simulink model "Torque_Control_ETR07"  (R2017b)
settings: Solver=FixedStepAuto  StartTime=0.0  StopTime=10.0  RelTol=1e-3
libraries: simulink x15, dspstat3 x1
(part 1 of 5)
settings Model: Creator=cspt  LastModifiedBy=cspt
settings RTWCC: SystemTargetFile=irt.tlc  TemplateMakefile=irt_default_tmf  Description=INTECRIO Real-Time Target
settings STFCustomTargetCC: TargetLangStandard=C99 (ISO)  UtilityFuncGeneration=Shared location  SystemTargetFile=irt.tlc
settings GRTTargetCC: UtilityFuncGeneration=Shared location  ParMdlRefBuildCompliant=off  CompOptLevelCompliant=off  ConcurrentExecutionCompliant=off  CombineOutputUpdateFcns=off  MatFileLogging=off  CPPClassGenCompliant=off  GRTInterface=on  UseToolchainInfoCompliant=off  GenerateASAP2=on

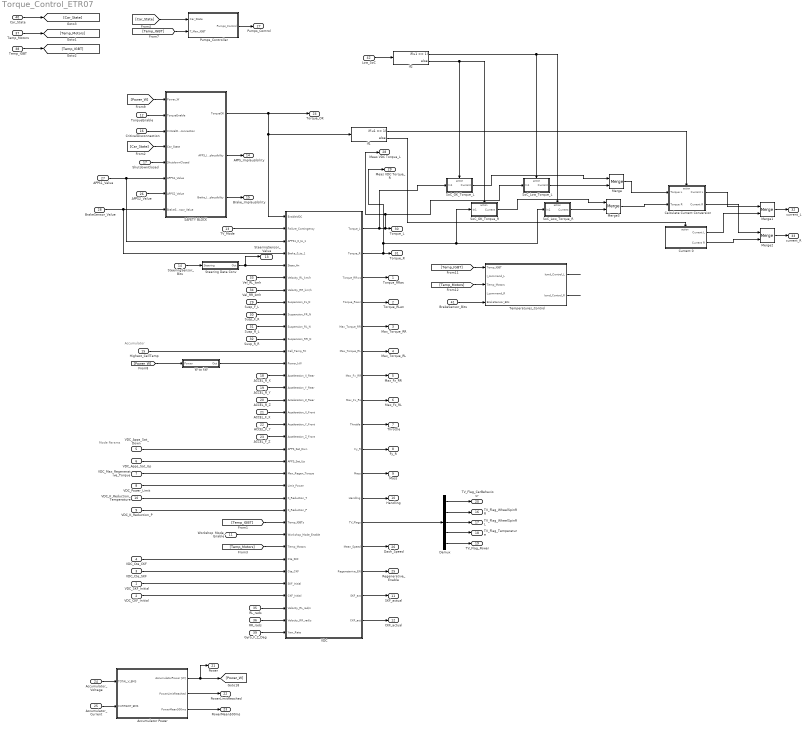
== system Torque_Control_ETR07 ==
  note: Mode Params
  note: Accumulator
  VDC_SKF_Initial : Inport
  VDC_CKF_Initial : Inport  Port=2
  VDC_Cte_SKF : Inport  Port=3
  VDC_Cte_CKF : Inport  Port=4
  VDC_Apps_Sat_Down : Inport  Port=5
  VDC_Apps_Sat_Up : Inport  Port=6
  VDC_Max_Regenerative_Torque : Inport  Port=7
  VDC_Power_Limit : Inport  Port=8
  VDC_K_Reduction_P : Inport  Port=9
  VDC_K_Reduction_Temperature : Inport  Port=10
  Workshop_Mode_Enable : Inport  Port=11
  TorqueEnable : Inport  Port=12
  TV_Mode : Inport  Port=13
  SteeringSensor_Bits : Inport  Port=14
  Highest_CellTemp : Inport  Port=15
  CriticalDisconnection : Inport  Port=16
  ShutdownClosed : Inport  Port=17
  ACCEL_R_X : Inport  Port=18
  ACCEL_R_Y : Inport  Port=19
  ACCEL_R_Z : Inport  Port=20
  ACCEL_F_X : Inport  Port=21
  ACCEL_F_Y : Inport  Port=22
  ACCEL_F_Z : Inport  Port=23
  Accumulator_Voltage : Inport  Port=24
  Accumulator_Current : Inport  Port=25
  APPS2_Value : Inport  Port=26
  APPS1_Value : Inport  Port=27
  BrakeSensor_Value : Inport  Port=28
  Susp_F_L : Inport  Port=29
  Susp_F_R : Inport  Port=30
  Susp_R_L : Inport  Port=31
  Susp_R_R : Inport  Port=32
  Vel_RL_kmh : Inport  Port=33
  Vel_RR_kmh : Inport  Port=34
  RL_rads : Inport  Port=35
  RR_rads : Inport  Port=36
  Temp_Motors : Inport  Port=37
  Temp_IGBT : Inport  Port=38
  Gyro_F_Z_Deg : Inport  Port=39
  Car_State : Inport  Port=40
  BrakeSensor_Bits : Inport  Port=41
  Low_SoC : Inport  Port=42
  Accumulator Power : Subsystem
  Calculate Current Conversion : Subsystem
  Current 0 : Subsystem  TreatAsAtomicUnit=on
  Demux : Demux  Outputs=5
  If1 : If  IfExpression=u1 == 1
  If2 : If  IfExpression=u1 == 1
  Merge{,1..3} (4 alike) : Merge
  Pumps_Controller : Subsystem
  SAFETY BLOCK : Subsystem
  SoC_Low_Torque_L : Subsystem  TreatAsAtomicUnit=on
  SoC_Low_Torque_R : Subsystem  TreatAsAtomicUnit=on
  SoC_OK_Torque_L : Subsystem  TreatAsAtomicUnit=on
  SoC_OK_Torque_R : Subsystem  TreatAsAtomicUnit=on
  Steering Data Conv : Subsystem
  Temperatures_Control : Subsystem
  VDC : Subsystem
  W to kW : Subsystem
  Torque_RRwc : Outport
  Torque_RLwc : Outport  Port=2
  Max_Torque_RR : Outport  Port=3
  Max_Torque_RL : Outport  Port=4
  Max_Fx_RR : Outport  Port=5
  Max_Fx_RL : Outport  Port=6
  Throttle : Outport  Port=7
  Fy_R : Outport  Port=8
  Mass : Outport  Port=9
  Handling : Outport  Port=10
  SKF_actual : Outport  Port=11
  CKF_actual : Outport  Port=12
  SteeringSensor_Value : Outport  Port=13
  APPS_Implausibility : Outport  Port=14
  Brake_Implausibility : Outport  Port=15
  TV_Flag_WheelSpinRR : Outport  Port=16
  TV_Flag_WheelSpinRL : Outport  Port=17
  TV_Flag_Temperature : Outport  Port=18
  TV_Flag_Power : Outport  Port=19
  TV_Flag_CarBehaviour : Outport  Port=20
  Power : Outport  Port=21
  PowerLimitReached : Outport  Port=22
  PowerMean500ms : Outport  Port=23
  Torque_OK : Outport  Port=24
  Regenerative_Enable : Outport  Port=25
  Dash_Speed : Outport  Port=26
  Pumps_Control : Outport  Port=27
  Meas VDC Torque_L : Outport  Port=28
  Meas VDC Torque_R : Outport  Port=29
  Torque_L : Outport  Port=30
  Torque_R : Outport  Port=31
  current_L : Outport  Port=32
  current_R : Outport  Port=33
  wires:
  Current 0/2(Current R) -> Merge2/2
  Accumulator Power/1(AccumulatorPower [W]) -> [Power_W], Power/1
  VDC_K_Reduction_P/1 -> VDC/25(K_Reduction_P)
  Workshop_Mode_Enable/1 -> VDC/27(Workshop_Mode_Enable)
  SAFETY BLOCK/2(APPS_Implausibility) -> APPS_Implausibility/1
  VDC_Cte_SKF/1 -> VDC/30(Cte_CKF)
  Calculate Current Conversion/2(Current R) -> Merge2/1
  Demux/4 -> TV_Flag_Temperature/1
  VDC_Apps_Sat_Down/1 -> VDC/20(APPS_Sat_Dwn)
  VDC_Max_Regenerative_Torque/1 -> VDC/22(Max_Regen_Torque)
  VDC_K_Reduction_Temperature/1 -> VDC/24(K_Reduction_T)
  VDC_Power_Limit/1 -> VDC/23(Limit_Power)
  VDC_Cte_CKF/1 -> VDC/29(Cte_SKF)
  VDC_SKF_Initial/1 -> VDC/31(SKF_Initial)
  VDC/2(Torque_R) -> SoC_OK_Torque_R/1(In1), SoC_Low_Torque_R/1(In1), Meas VDC Torque_R/1, Torque_R/1
  VDC/3(Torque_RRwc) -> Torque_RRwc/1
  TV_Mode/1 -> VDC/2(Failure_Contingency)
  W to kW/1(Out) -> VDC/13(Power_kW)
  Highest_CellTemp/1 -> VDC/12(Cell_Temp_ºC)
  ACCEL_F_X/1 -> VDC/17(Acceleration_X_Front)
  [Car_State] -> SAFETY BLOCK/4(Car_State)
  ACCEL_R_X/1 -> VDC/14(Acceleration_X_Rear)
  Accumulator_Current/1 -> Accumulator Power/2(CURRENT_BMS)
  Accumulator Power/3(PowerMean500ms) -> PowerMean500ms/1
  SteeringSensor_Bits/1 -> Steering Data Conv/1("Steering ")
  [Temp_Motors] -> VDC/28(Temp_Motors)
  [Temp_IGBT] -> Pumps_Controller/2(T_Max_IGBT)
  VDC/14(Mean_Speed) -> Dash_Speed/1
  Pumps_Controller/1(Pumps_Control) -> Pumps_Control/1
  Demux/1 -> TV_Flag_CarBehaviour/1
  VDC/15(Regenetarive_EN) -> Regenerative_Enable/1
  VDC/10(Fy_R) -> Fy_R/1
  Current 0/1(Current L) -> Merge1/2
  Calculate Current Conversion/1(Current L) -> Merge1/1
  If1/2 -> Current 0/Action
  If1/1 -> Calculate Current Conversion/Action
  VDC_Apps_Sat_Up/1 -> VDC/21(APPS_Sat_Up)
  TorqueEnable/1 -> SAFETY BLOCK/2(TorqueEnable)
  VDC/5(Max_Torque_RR) -> Max_Torque_RR/1
  Accumulator_Voltage/1 -> Accumulator Power/1(TOTAL_V_BMS)
  Accumulator Power/2(PowerLimitReached) -> PowerLimitReached/1
  VDC/7(Max_Fx_RR) -> Max_Fx_RR/1
  VDC/8(Max_Fx_RL) -> Max_Fx_RL/1
  VDC_CKF_Initial/1 -> VDC/32(CKF_Initial)
  SAFETY BLOCK/3(Brake_Implausibility) -> Brake_Implausibility/1
  Demux/2 -> TV_Flag_WheelSpinRR/1
  ACCEL_R_Y/1 -> VDC/15(Acceleration_Y_Rear)
  ACCEL_R_Z/1 -> VDC/16(Acceleration_Z_Rear)
  Demux/5 -> TV_Flag_Power/1
  VDC/9(Throttle) -> Throttle/1
  Demux/3 -> TV_Flag_WheelSpinRL/1
  ACCEL_F_Z/1 -> VDC/19(Acceleration_Z_Front)
  [Power_W] -> W to kW/1(Power)
  [Temp_IGBT] -> VDC/26(Temp_IGBTs)
  ACCEL_F_Y/1 -> VDC/18(Acceleration_Y_Front)
  CriticalDisconnection/1 -> SAFETY BLOCK/3(CriticalDisconnection)
  SAFETY BLOCK/1(TorqueOK) -> Torque_OK/1, VDC/1(EnableVDC), If1/1
  ShutdownClosed/1 -> SAFETY BLOCK/5(ShutdownClosed)
  VDC/11(Mass) -> Mass/1
  VDC/17(CKF_act) -> CKF_actual/1
  VDC/12(Handling) -> Handling/1
  VDC/13(TV_Flags) -> Demux/1
  VDC/6(Max_Torque_RL) -> Max_Torque_RL/1
  VDC/16(SKF_act) -> SKF_actual/1
  [Power_W] -> SAFETY BLOCK/1(Power_W)
  VDC/4(Torque_RLwc) -> Torque_RLwc/1
  APPS1_Value/1 -> SAFETY BLOCK/6(APPS1_Value), VDC/3(APPS1_0_to_1)
  BrakeSensor_Value/1 -> VDC/4(Brake_0_to_1), SAFETY BLOCK/8(BrakeSensor_Value)
  Susp_F_L/1 -> VDC/8(Suspension_FL_N)
  Susp_F_R/1 -> VDC/9(Suspension_FR_N)
  Susp_R_L/1 -> VDC/10(Suspension_RL_N)
  Susp_R_R/1 -> VDC/11(Suspension_RR_N)
  Temp_Motors/1 -> [Temp_Motors]
  Temp_IGBT/1 -> [Temp_IGBT]
  APPS2_Value/1 -> SAFETY BLOCK/7(APPS2_Value)
  Gyro_F_Z_Deg/1 -> VDC/35(Yaw_Rate)
  Car_State/1 -> [Car_State]
  [Car_State] -> Pumps_Controller/1(Car_State)
  Steering Data Conv/1(Out) -> SteeringSensor_Value/1, VDC/5(Steer_An)
  Vel_RR_kmh/1 -> VDC/7(Velocity_RR_km/h)
  Vel_RL_kmh/1 -> VDC/6(Velocity_RL_km/h)
  RL_rads/1 -> VDC/33(Velocity_RL_rad/s)
  RR_rads/1 -> VDC/34(Velocity_RR_rad/s)
  VDC/1(Torque_L) -> SoC_OK_Torque_L/1(In1), SoC_Low_Torque_L/1(In1), Meas VDC Torque_L/1, Torque_L/1
  Merge1/1 -> current_L/1
  Merge2/1 -> current_R/1
  [Temp_IGBT] -> Temperatures_Control/1(Temp_IGBT)
  [Temp_Motors] -> Temperatures_Control/3("Temp_Motors ")
  Temperatures_Control/2(Icmd_Control_R) -> ?
  Temperatures_Control/1("Icmd_Control_L ") -> ?
  BrakeSensor_Bits/1 -> Temperatures_Control/5(BrakeSensor_Bits)
  Low_SoC/1 -> If2/1
  If2/2 -> SoC_OK_Torque_R/Action, SoC_OK_Torque_L/Action
  If2/1 -> SoC_Low_Torque_L/Action, SoC_Low_Torque_R/Action
  Merge3/1 -> Calculate Current Conversion/2(Torque R)
  Merge/1 -> Calculate Current Conversion/1(Torque L)
  SoC_Low_Torque_R/1(Current) -> Merge3/2
  SoC_OK_Torque_R/1(Current) -> Merge3/1
  SoC_Low_Torque_L/1(Current) -> Merge/2
  SoC_OK_Torque_L/1(Current) -> Merge/1

== system Torque_Control_ETR07/Accumulator Power ==
  TOTAL_V_BMS : Inport
  CURRENT_BMS : Inport  Port=2
  PowerLimitDetection : Subsystem  TreatAsAtomicUnit=on
  Product : Product
  AccumulatorPower [W] : Outport
  PowerLimitReached : Outport  Port=2
  PowerMean500ms : Outport  Port=3
  wires:
  CURRENT_BMS/1 -> Product/2
  Product/1 -> AccumulatorPower [W]/1, PowerLimitDetection/1(Power)
  PowerLimitDetection/1(PowerLimitReached) -> PowerLimitReached/1
  PowerLimitDetection/2(PowerMean500ms) -> PowerMean500ms/1
  TOTAL_V_BMS/1 -> Product/1

== system Torque_Control_ETR07/Calculate Current Conversion ==
  Torque L : Inport
  Torque R : Inport  Port=2
  Action Port : ActionPort  ActionType=then
  Gain : Gain  Gain=-1
  KT_L_TORKY : Subsystem  TreatAsAtomicUnit=on
  KT_R_EMY : Subsystem  TreatAsAtomicUnit=on
  Current L : Outport
  Current R : Outport  Port=2
  wires:
  Torque R/1 -> KT_R_EMY/1(Torque)
  KT_L_TORKY/1(Current) -> Gain/1
  KT_R_EMY/1(Current) -> Current R/1
  Torque L/1 -> KT_L_TORKY/1(Torque)
  Gain/1 -> Current L/1

== system Torque_Control_ETR07/Current 0 ==
  Action Port : ActionPort  ActionType=else
  Constant : Constant  Value=0
  Current L : Outport
  Current R : Outport  Port=2
  wires:
  Constant/1 -> Current R/1, Current L/1

== system Torque_Control_ETR07/Pumps_Controller ==
  note: if car is in rtd or temperature of igbt is more than 50 degrees
  Car_State : Inport
  T_Max_IGBT : Inport  Port=2
  Compare To Constant : simulink/Logic and Bit Operations/Compare To Constant  relop=>  const=50  OutDataTypeStr=boolean
  Compare To Constant1 : simulink/Logic and Bit Operations/Compare To Constant  relop===  const=15  OutDataTypeStr=boolean
  DocBlock1 : simulink/Model-Wide Utilities/DocBlock  DocumentType=Text
      content=|
      | Aquest mòdul activa les bombes sempre que:
      | o bé s'està conduint
      | o bé la temperatura dels igbts de l'inversor supera 50 graus
  If : If  IfExpression=u1 == 1
  Logical Operator : Logic  Operator=OR  AllPortsSameDT=off  OutDataTypeStr=boolean
  Merge : Merge
  Pumps_Control_OFF : Subsystem  TreatAsAtomicUnit=on
  Pumps_Control_ON : Subsystem  TreatAsAtomicUnit=on
  Pumps_Control : Outport
  wires:
  Pumps_Control_OFF/1(0) -> Merge/2
  Car_State/1 -> Compare To Constant1/1
  If/2 -> Pumps_Control_OFF/Action
  If/1 -> Pumps_Control_ON/Action
  Pumps_Control_ON/1(1) -> Merge/1
  T_Max_IGBT/1 -> Compare To Constant/1
  Merge/1 -> Pumps_Control/1
  Logical Operator/1 -> If/1
  Compare To Constant/1 -> Logical Operator/2
  Compare To Constant1/1 -> Logical Operator/1

== system Torque_Control_ETR07/SAFETY BLOCK ==
  note: CriticalDisconnection -> 1
      | OK -> 0
  Power_W : Inport
  TorqueEnable : Inport  Port=2
  CriticalDisconnection : Inport  Port=3
  Car_State : Inport  Port=4
  ShutdownClosed : Inport  Port=5
  APPS1_Value : Inport  Port=6
  APPS2_Value : Inport  Port=7
  BrakeSensor_Value : Inport  Port=8
  APPS_IMPLAUSIBILITY : Subsystem
  BRAKE_IMPLAUSIBILITY : Subsystem
  Compare To Constant : simulink/Logic and Bit Operations/Compare To Constant  relop===  const=15  OutDataTypeStr=boolean
  Logical Operator : Logic  Inputs=7  OutDataTypeStr=boolean
  Logical Operator1 : Logic  Operator=NOT  IconShape=distinctive  AllPortsSameDT=off  OutDataTypeStr=boolean
  Logical Operator2 : Logic  Operator=NOT  IconShape=distinctive  AllPortsSameDT=off  OutDataTypeStr=boolean
  NOT : Logic  Operator=NOT  IconShape=distinctive  AllPortsSameDT=off  OutDataTypeStr=boolean
  "Power is under 100kW " : simulink/Logic and Bit Operations/Compare To Constant  relop=<  const=100000  OutDataTypeStr=boolean
  TorqueOK : Outport
  APPS_Implausibility : Outport  Port=2
  Brake_Implausibility : Outport  Port=3
  wires:
  Logical Operator/1 -> TorqueOK/1
  ShutdownClosed/1 -> Logical Operator/7
  Car_State/1 -> Compare To Constant/1
  NOT/1 -> Logical Operator/3
  CriticalDisconnection/1 -> NOT/1
  TorqueEnable/1 -> Logical Operator/2
  Power_W/1 -> "Power is under 100kW "/1
  "Power is under 100kW "/1 -> Logical Operator/1
  BrakeSensor_Value/1 -> BRAKE_IMPLAUSIBILITY/3(BrakeSensor_Value)
  APPS2_Value/1 -> BRAKE_IMPLAUSIBILITY/2(APPS2_Value), APPS_IMPLAUSIBILITY/2(APPS2)
  APPS1_Value/1 -> BRAKE_IMPLAUSIBILITY/1(APPS1_Value), APPS_IMPLAUSIBILITY/1(APPS1)
  APPS_IMPLAUSIBILITY/1(OK) -> Logical Operator/5, Logical Operator1/1
  BRAKE_IMPLAUSIBILITY/1(OK_BRS) -> Logical Operator/6, Logical Operator2/1
  Logical Operator2/1 -> Brake_Implausibility/1
  Logical Operator1/1 -> APPS_Implausibility/1
  Compare To Constant/1 -> Logical Operator/4

== system Torque_Control_ETR07/SoC_Low_Torque_L ==
  In1 : Inport
  Action Port : ActionPort  ActionType=then
  Constant : Constant  Value=5
  Divide : Product  Inputs=*/
  Saturation : Saturate  UpperLimit=30  LowerLimit=0
  Current : Outport
  wires:
  In1/1 -> Divide/1
  Constant/1 -> Divide/2
  Divide/1 -> Saturation/1
  Saturation/1 -> Current/1

== system Torque_Control_ETR07/SoC_Low_Torque_R ==
  In1 : Inport
  Action Port : ActionPort  ActionType=then
  Constant : Constant  Value=5
  Divide : Product  Inputs=*/
  Saturation : Saturate  UpperLimit=30  LowerLimit=0
  Current : Outport
  wires:
  In1/1 -> Divide/1
  Constant/1 -> Divide/2
  Divide/1 -> Saturation/1
  Saturation/1 -> Current/1

== system Torque_Control_ETR07/SoC_OK_Torque_L ==
  In1 : Inport
  Action Port : ActionPort  ActionType=else
  Current : Outport
  wires:
  In1/1 -> Current/1

== system Torque_Control_ETR07/SoC_OK_Torque_R ==
  In1 : Inport
  Action Port : ActionPort  ActionType=else
  Current : Outport
  wires:
  In1/1 -> Current/1

== system Torque_Control_ETR07/Steering Data Conv ==
  "Steering " : Inport
  Divide : Product  Inputs=**/
  Gain : Gain  Gain=115
  Low Pass : Subsystem  TreatAsAtomicUnit=on
  Sum : Sum  Inputs=|+-
  half range : Constant  Value=2
  range : Constant  Value=407
  zero : Constant  Value=222
  Out : Outport
  wires:
  zero/1 -> Sum/2
  Sum/1 -> Divide/1
  Divide/1 -> Gain/1
  range/1 -> Divide/3
  half range/1 -> Divide/2
  "Steering "/1 -> Sum/1
  Gain/1 -> Low Pass/1(IN)
  Low Pass/1(OUT) -> Out/1

== system Torque_Control_ETR07/Temperatures_Control ==
  Temp_IGBT : Inport
  I_command_L : Inport  Port=2
  "Temp_Motors " : Inport  Port=3
  "I_command_R " : Inport  Port=4
  BrakeSensor_Bits : Inport  Port=5
  Gain : Gain  Gain=0.75
  Gain1 : Gain  Gain=0.75
  If : If  NumInputs=2  IfExpression=u2 > u1
  If Action Subsystem : Subsystem  TreatAsAtomicUnit=on
  If Action Subsystem1 : Subsystem  TreatAsAtomicUnit=on
  If Action Subsystem2 : Subsystem  TreatAsAtomicUnit=on
  If Action Subsystem3 : Subsystem  TreatAsAtomicUnit=on
  If1 : If  NumInputs=2  IfExpression=u2 > u1
  MATLAB Function2 : MATLAB Function  TreatAsAtomicUnit=on
  Max_T_IGBT : Constant  Value=80
  "Max_T_Motor " : Constant  Value=150
  Merge : Merge
  Merge1 : Merge
  cte_1 : Constant  Value=100
  cte_2 : Constant  Value=150
  "Icmd_Control_L " : Outport
  Icmd_Control_R : Outport  Port=2
  wires:
  Temp_IGBT/1 -> If/2
  Max_T_IGBT/1 -> Gain/1
  Gain/1 -> If/1
  If Action Subsystem1/1(Ok) -> Merge/2
  If Action Subsystem/1(Problema) -> Merge/1
  If/1 -> If Action Subsystem/Action
  If/2 -> If Action Subsystem1/Action
  "Max_T_Motor "/1 -> Gain1/1
  Gain1/1 -> If1/1
  "Temp_Motors "/1 -> If1/2
  If1/2 -> If Action Subsystem3/Action
  If1/1 -> If Action Subsystem2/Action
  If Action Subsystem3/1(OK) -> Merge1/2
  If Action Subsystem2/1(Problema) -> Merge1/1
  I_command_L/1 -> MATLAB Function2/4(I_command_L)
  Merge1/1 -> MATLAB Function2/6(T_motor)
  Merge/1 -> MATLAB Function2/3(T_IGBT)
  MATLAB Function2/1(I_cmd_L) -> "Icmd_Control_L "/1
  cte_1/1 -> MATLAB Function2/1(cte_1)
  cte_2/1 -> MATLAB Function2/2(cte_2)
  "I_command_R "/1 -> MATLAB Function2/5(I_command_R)
  MATLAB Function2/2(I_cmd_R) -> Icmd_Control_R/1
  BrakeSensor_Bits/1 -> MATLAB Function2/7(BrakeSensor)

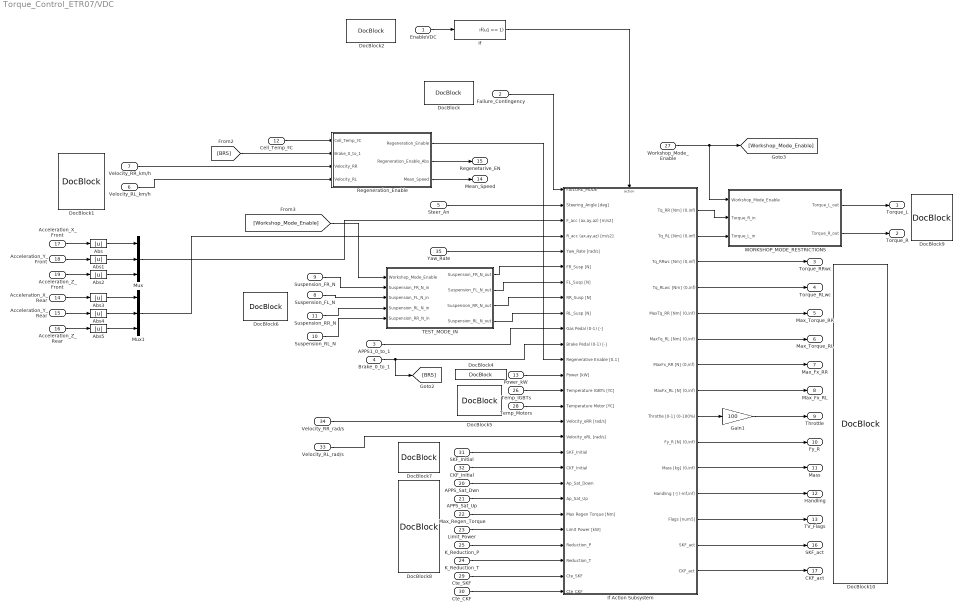
== system Torque_Control_ETR07/VDC ==
  EnableVDC : Inport
  Failure_Contingency : Inport  Port=2
  APPS1_0_to_1 : Inport  Port=3
  Brake_0_to_1 : Inport  Port=4
  Steer_An : Inport  Port=5
  Velocity_RL_km/h : Inport  Port=6
  Velocity_RR_km/h : Inport  Port=7
  Suspension_FL_N : Inport  Port=8
  Suspension_FR_N : Inport  Port=9
  Suspension_RL_N : Inport  Port=10
  Suspension_RR_N : Inport  Port=11
  Cell_Temp_ºC : Inport  Port=12
  Power_kW : Inport  Port=13
  Acceleration_X_Rear : Inport  Port=14
  Acceleration_Y_Rear : Inport  Port=15
  Acceleration_Z_Rear : Inport  Port=16
  Acceleration_X_Front : Inport  Port=17
  Acceleration_Y_Front : Inport  Port=18
  Acceleration_Z_Front : Inport  Port=19
  APPS_Sat_Dwn : Inport  Port=20
  APPS_Sat_Up : Inport  Port=21
  Max_Regen_Torque : Inport  Port=22
  Limit_Power : Inport  Port=23
  K_Reduction_T : Inport  Port=24
  K_Reduction_P : Inport  Port=25
  Temp_IGBTs : Inport  Port=26
  Workshop_Mode_Enable : Inport  Port=27
  Temp_Motors : Inport  Port=28
  Cte_SKF : Inport  Port=29
  Cte_CKF : Inport  Port=30
  SKF_Initial : Inport  Port=31
  CKF_Initial : Inport  Port=32
  Velocity_RL_rad/s : Inport  Port=33
  Velocity_RR_rad/s : Inport  Port=34
  Yaw_Rate : Inport  Port=35
  Abs{,1..5} (6 alike) : Abs
  DocBlock{,1..2,4..10} (10 alike) : simulink/Model-Wide Utilities/DocBlock  DocumentType=Text
  Gain1 : Gain  Gain=100
  If : If  IfExpression=u1 == 1  ShowElse=off
  If Action Subsystem : Subsystem  TreatAsAtomicUnit=on
  Mux : Mux  Inputs=3
  Mux1 : Mux  Inputs=3
  Regeneration_Enable : Subsystem  TreatAsAtomicUnit=on
  TEST_MODE_IN : Subsystem  TreatAsAtomicUnit=on
  WORKSHOP_MODE_RESTRICTIONS : Subsystem  TreatAsAtomicUnit=on
  Torque_L : Outport
  Torque_R : Outport  Port=2
  Torque_RRwc : Outport  Port=3
  Torque_RLwc : Outport  Port=4
  Max_Torque_RR : Outport  Port=5
  Max_Torque_RL : Outport  Port=6
  Max_Fx_RR : Outport  Port=7
  Max_Fx_RL : Outport  Port=8
  Throttle : Outport  Port=9
  Fy_R : Outport  Port=10
  Mass : Outport  Port=11
  Handling : Outport  Port=12
  TV_Flags : Outport  Port=13
  Mean_Speed : Outport  Port=14
  Regenetarive_EN : Outport  Port=15
  SKF_act : Outport  Port=16
  CKF_act : Outport  Port=17
  wires:
  SKF_Initial/1 -> If Action Subsystem/18(SKF_Initial)
  Regeneration_Enable/2(Regeneration_Enable_Abs) -> Regenetarive_EN/1
  Velocity_RR_km/h/1 -> Regeneration_Enable/3(Velocity_RR)
  Acceleration_Z_Front/1 -> Abs2/1
  Abs2/1 -> Mux/3
  Gain1/1 -> Throttle/1
  If Action Subsystem/7(MaxFx_RR [N] (0,inf)) -> Max_Fx_RR/1
  If Action Subsystem/6(MaxTq_RL [Nm] (0,inf)) -> Max_Torque_RL/1
  TEST_MODE_IN/4(Suspension_RL_N_out) -> If Action Subsystem/9(RL_Susp [N])
  Acceleration_X_Rear/1 -> Abs3/1
  Acceleration_Y_Front/1 -> Abs1/1
  TEST_MODE_IN/2(Suspension_FL_N_out) -> If Action Subsystem/7(FL_Susp [N])
  Abs4/1 -> Mux1/2
  If Action Subsystem/8(MaxFx_RL [N] (0,inf)) -> Max_Fx_RL/1
  Max_Regen_Torque/1 -> If Action Subsystem/22(Max Regen Torque [Nm])
  Power_kW/1 -> If Action Subsystem/13(Power [kW])
  If Action Subsystem/1(Tq_RR [Nm] (0,inf)) -> WORKSHOP_MODE_RESTRICTIONS/2(Torque_R_in)
  Cte_CKF/1 -> If Action Subsystem/27(Cte_CKF)
  Abs/1 -> Mux/1
  Abs5/1 -> Mux1/3
  WORKSHOP_MODE_RESTRICTIONS/2(Torque_R_out) -> Torque_R/1
  Acceleration_Y_Rear/1 -> Abs4/1
  APPS_Sat_Up/1 -> If Action Subsystem/21(Ap_Sat_Up)
  CKF_Initial/1 -> If Action Subsystem/19(CKF_Initial)
  WORKSHOP_MODE_RESTRICTIONS/1(Torque_L_out) -> Torque_L/1
  Acceleration_Z_Rear/1 -> Abs5/1
  If Action Subsystem/3(Tq_RRwc [Nm] (0,inf)) -> Torque_RRwc/1
  Temp_IGBTs/1 -> If Action Subsystem/14(Temperature IGBTs [ºC])
  Regeneration_Enable/1(Regeneration_Enable) -> If Action Subsystem/12(Regenerative Enable [0,1])
  Suspension_FL_N/1 -> TEST_MODE_IN/3(Suspension_FL_N_in)
  Suspension_FR_N/1 -> TEST_MODE_IN/2(Suspension_FR_N_in)
  TEST_MODE_IN/1(Suspension_FR_N_out) -> If Action Subsystem/6(FR_Susp [N])
  K_Reduction_T/1 -> If Action Subsystem/25(Reduction_T)
  Velocity_RR_rad/s/1 -> If Action Subsystem/16(Velocity_eRR [rad/s])
  Limit_Power/1 -> If Action Subsystem/23(Limit Power [kW])
  If Action Subsystem/14(SKF_act) -> SKF_act/1
  [BRS] -> Regeneration_Enable/2(Brake_0_to_1)
  APPS1_0_to_1/1 -> If Action Subsystem/10(Gas Pedal (0-1) [-])
  If Action Subsystem/4(Tq_RLwc [Nm] (0,inf)) -> Torque_RLwc/1
  If Action Subsystem/5(MaxTq_RR [Nm] (0,inf)) -> Max_Torque_RR/1
  Brake_0_to_1/1 -> If Action Subsystem/11(Brake Pedal (0-1) [-]), [BRS]
  Cte_SKF/1 -> If Action Subsystem/26(Cte_SKF)
  Velocity_RL_km/h/1 -> Regeneration_Enable/4(Velocity_RL)
  If Action Subsystem/11(Mass [kg] (0,inf)) -> Mass/1
  Temp_Motors/1 -> If Action Subsystem/15(Temperature Motor [ºC])
  If Action Subsystem/9(Throttle [0-1] (0-100%)) -> Gain1/1
  If Action Subsystem/2(Tq_RL [Nm] (0,inf)) -> WORKSHOP_MODE_RESTRICTIONS/3(Torque_L_in)
  Velocity_RL_rad/s/1 -> If Action Subsystem/17(Velocity_eRL [rad/s])
  EnableVDC/1 -> If/1
  K_Reduction_P/1 -> If Action Subsystem/24(Reduction_P)
  Regeneration_Enable/3(Mean_Speed) -> Mean_Speed/1
  Suspension_RL_N/1 -> TEST_MODE_IN/5(Suspension_RR_N_in)
  APPS_Sat_Dwn/1 -> If Action Subsystem/20(Ap_Sat_Down)
  If Action Subsystem/10(Fy_R [N] (0,inf)) -> Fy_R/1
  If Action Subsystem/13(Flags [num5]) -> TV_Flags/1
  Abs1/1 -> Mux/2
  [Workshop_Mode_Enable] -> TEST_MODE_IN/1(Workshop_Mode_Enable)
  Acceleration_X_Front/1 -> Abs/1
  Abs3/1 -> Mux1/1
  Suspension_RR_N/1 -> TEST_MODE_IN/4(Suspension_RL_N_in)
  If Action Subsystem/12(Handling [-] (-inf,inf)) -> Handling/1
  TEST_MODE_IN/3(Suspension_RR_N_out) -> If Action Subsystem/8(RR_Susp [N])
  Cell_Temp_ºC/1 -> Regeneration_Enable/1(Cell_Temp_ºC)
  Workshop_Mode_Enable/1 -> WORKSHOP_MODE_RESTRICTIONS/1(Workshop_Mode_Enable), [Workshop_Mode_Enable]
  If Action Subsystem/15(CKF_act) -> CKF_act/1
  Steer_An/1 -> If Action Subsystem/2(Steering_Angle [deg])
  Mux/1 -> If Action Subsystem/3(F_acc (ax,ay,az) [m/s2])
  Mux1/1 -> If Action Subsystem/4(R_acc (ax,ay,az) [m/s2])
  Failure_Contingency/1 -> If Action Subsystem/1(FAILURE_MODE)
  Yaw_Rate/1 -> If Action Subsystem/5(Yaw_Rate [rad/s])
  If/1 -> If Action Subsystem/Action

== system Torque_Control_ETR07/W to kW ==
  Power : Inport
  0-100 to 0-2 : Constant  Value=1000
  Divide5 : Product  Inputs=*/
  Out : Outport
  wires:
  Power/1 -> Divide5/1
  0-100 to 0-2/1 -> Divide5/2
  Divide5/1 -> Out/1

== system Torque_Control_ETR07/Accumulator Power/PowerLimitDetection ==
  note: mean:500ms
      | time:25ms
      | moving window: 500/25=20
  Power : Inport
  Data Store Memory10 : DataStoreMemory  ReadBeforeWriteMsg=warning  WriteAfterWriteMsg=warning  WriteAfterReadMsg=warning  ShowAdditionalParam=off
  Data Store Read30 : DataStoreRead
  Data Store Write20 : DataStoreWrite
  If : If  IfExpression=u1 >= 80000
  LimitReached : Subsystem  TreatAsAtomicUnit=on
  Merge1 : Merge
  Moving Average : dspstat3/Moving Average  Method=Sliding window  SpecifyWindowLength=on  WindowLength=20  ForgettingFactor=0.9  SimulateUsing=Code generation
  OK_OrLatch : Subsystem  TreatAsAtomicUnit=on
  PowerLimitReached : Outport
  PowerMean500ms : Outport  Port=2
  wires:
  Power/1 -> Moving Average/1
  Moving Average/1 -> If/1, PowerMean500ms/1
  If/1 -> LimitReached/Action
  If/2 -> OK_OrLatch/Action
  LimitReached/1("Out ") -> Merge1/1
  OK_OrLatch/1(Out 1) -> Merge1/2
  Merge1/1 -> Data Store Write20/1, PowerLimitReached/1
  Data Store Read30/1 -> OK_OrLatch/1(IN)

== system Torque_Control_ETR07/Calculate Current Conversion/KT_L_TORKY ==
  Torque : Inport
  A : Constant  Value=0.002359
  Add : Sum  Inputs=+++
  B : Constant  Value=1.0396
  Bypass : Subsystem  TreatAsAtomicUnit=on
  Bypass_Torque : Subsystem  TreatAsAtomicUnit=on
  C : Constant  Value=6.363
  If : If  IfExpression=u1 == 0
  If1 : If  IfExpression=u1 >=0
  Is_Zero : Subsystem  TreatAsAtomicUnit=on
  Math Function : Math  Operator=square  SaturateOnIntegerOverflow=on
  Merge : Merge
  Merge1 : Merge
  Merge2 : Merge
  Negative : Subsystem  TreatAsAtomicUnit=on
  Product : Product
  Product1 : Product
  Zero : Constant  Value=0
  Current : Outport
  wires:
  Product/1 -> Add/1
  Product1/1 -> Add/2
  B/1 -> Product1/2
  Math Function/1 -> Product/1
  Add/1 -> Bypass_Torque/1(In1)
  Zero/1 -> Is_Zero/1(In1)
  Bypass_Torque/1(Out1) -> Merge/1
  Is_Zero/1(Out1) -> Merge/2
  Merge/1 -> Current/1
  If/2 -> Bypass_Torque/Action
  If/1 -> Is_Zero/Action
  Torque/1 -> Product1/1, Math Function/1, If/1, If1/1
  A/1 -> Negative/1(In1), Bypass/1(In1)
  C/1 -> Negative/2(In2), Bypass/2(In2)
  If1/1 -> Bypass/Action
  If1/2 -> Negative/Action
  Bypass/1(Out1) -> Merge1/1
  Bypass/2(Out2) -> Merge2/1
  Negative/1(Out1) -> Merge1/2
  Negative/2(Out2) -> Merge2/2
  Merge1/1 -> Product/2
  Merge2/1 -> Add/3

== system Torque_Control_ETR07/Calculate Current Conversion/KT_R_EMY ==
  Torque : Inport
  A1 : Constant  Value=0.0030128
  Add : Sum  Inputs=+++
  B1 : Constant  Value=1.0388
  Bypass : Subsystem  TreatAsAtomicUnit=on
  Bypass_Torque : Subsystem  TreatAsAtomicUnit=on
  C1 : Constant  Value=6.5613
  If : If  IfExpression=u1 == 0
  If1 : If  IfExpression=u1 >=0
  Is_Zero : Subsystem  TreatAsAtomicUnit=on
  Math Function : Math  Operator=square  SaturateOnIntegerOverflow=on
  Merge : Merge
  Merge1 : Merge
  Merge2 : Merge
  Negative : Subsystem  TreatAsAtomicUnit=on
  Product : Product
  Product1 : Product
  Zero : Constant  Value=0
  Current : Outport
  wires:
  Product/1 -> Add/1
  Product1/1 -> Add/2
  B1/1 -> Product1/2
  Math Function/1 -> Product/1
  Add/1 -> Bypass_Torque/1(In1)
  Zero/1 -> Is_Zero/1(In1)
  Bypass_Torque/1(Out1) -> Merge/1
  Is_Zero/1(Out1) -> Merge/2
  Merge/1 -> Current/1
  If/2 -> Bypass_Torque/Action
  If/1 -> Is_Zero/Action
  Torque/1 -> Product1/1, Math Function/1, If/1, If1/1
  A1/1 -> Negative/1(In1), Bypass/1(In1)
  C1/1 -> Negative/2(In2), Bypass/2(In2)
  If1/1 -> Bypass/Action
  If1/2 -> Negative/Action
  Bypass/1(Out1) -> Merge1/1
  Bypass/2(Out2) -> Merge2/1
  Negative/1(Out1) -> Merge1/2
  Negative/2(Out2) -> Merge2/2
  Merge1/1 -> Product/2
  Merge2/1 -> Add/3

== system Torque_Control_ETR07/Pumps_Controller/Pumps_Control_OFF ==
  Action Port : ActionPort  ActionType=else
  Constant : Constant  Value=0
  0 : Outport
  wires:
  Constant/1 -> 0/1

== system Torque_Control_ETR07/Pumps_Controller/Pumps_Control_ON ==
  Action Port : ActionPort  ActionType=then
  Constant : Constant
  1 : Outport
  wires:
  Constant/1 -> 1/1

== system Torque_Control_ETR07/SAFETY BLOCK/APPS_IMPLAUSIBILITY ==
  APPS1 : Inport
  APPS2 : Inport  Port=2
  Ab : Abs
  If : If  IfExpression=u1 > 0.1
  Imp : Subsystem  TreatAsAtomicUnit=on
  Merge : Merge
  Not Imp : Subsystem  TreatAsAtomicUnit=on
  Sum : Sum  Inputs=|+-
  OK : Outport
  wires:
  APPS1/1 -> Sum/1
  APPS2/1 -> Sum/2
  Sum/1 -> Ab/1
  Ab/1 -> If/1
  Imp/1(Out1) -> Merge/1  "Bool 0"
  Not Imp/1(Out1) -> Merge/2  "Bool 1"
  Merge/1 -> OK/1
  If/2 -> Not Imp/Action
  If/1 -> Imp/Action

== system Torque_Control_ETR07/SAFETY BLOCK/BRAKE_IMPLAUSIBILITY ==
  APPS1_Value : Inport
  APPS2_Value : Inport  Port=2
  BrakeSensor_Value : Inport  Port=3
  Data Store Memory1 : DataStoreMemory  DataStoreName=AA  ReadBeforeWriteMsg=warning  WriteAfterWriteMsg=warning  WriteAfterReadMsg=warning  ShowAdditionalParam=off
  Data Store Read1 : DataStoreRead  DataStoreName=AA
  Data Store Write1 : DataStoreWrite  DataStoreName=AA
  If Action Subsystem2 : Subsystem  TreatAsAtomicUnit=on
  If Action Subsystem3 : Subsystem  TreatAsAtomicUnit=on
  If2 : If  NumInputs=3  IfExpression=(u1 > 0.25 & u3 > 0.25)|(u2 > 0.25 & u3 > 0.25)
  If3 : If  IfExpression=u1
  Imp Memo1 : Subsystem  TreatAsAtomicUnit=on
  Imp1 : Subsystem  TreatAsAtomicUnit=on
  Logical Operator1 : Logic  OutDataTypeStr=boolean
  MEMO1 : If  NumInputs=3  IfExpression=(u1 == 0 & u2 >0.05)|(u1 == 0 & u3 >0.05)
  Merge3 : Merge
  Merge4 : Merge
  Merge5 : Merge
  Not Imp Memo1 : Subsystem  TreatAsAtomicUnit=on
  Not Imp1 : Subsystem  TreatAsAtomicUnit=on
  OK_BRS : Outport
  wires:
  Imp Memo1/1(Out1) -> Merge4/1  "Bool 0"
  Data Store Read1/1 -> If3/1
  Merge5/1 -> MEMO1/1
  If3/1 -> If Action Subsystem2/Action
  If Action Subsystem3/1(Out1) -> Merge5/2
  Imp1/1(Out1) -> Merge3/1  "Bool 0"
  If3/2 -> If Action Subsystem3/Action
  Not Imp Memo1/1(Out1) -> Merge4/2  "Bool 1"
  Not Imp1/1(Out1) -> Merge3/2  "Bool 1"
  If2/2 -> Not Imp1/Action
  If2/1 -> Imp1/Action
  MEMO1/2 -> Not Imp Memo1/Action
  Merge3/1 -> Logical Operator1/1
  BrakeSensor_Value/1 -> If2/3
  APPS2_Value/1 -> MEMO1/3, If2/2
  MEMO1/1 -> Imp Memo1/Action
  If Action Subsystem2/1(Out1) -> Merge5/1
  Merge4/1 -> Logical Operator1/2
  APPS1_Value/1 -> MEMO1/2, If2/1
  Logical Operator1/1 -> OK_BRS/1, Data Store Write1/1

== system Torque_Control_ETR07/Steering Data Conv/Low Pass ==
  IN : Inport
  Data Store Memory : DataStoreMemory  DataStoreName=Previous_IN  ReadBeforeWriteMsg=warning  WriteAfterWriteMsg=warning  WriteAfterReadMsg=warning  ShowAdditionalParam=off
  Data Store Memory1 : DataStoreMemory  DataStoreName=Previous_OUT  ReadBeforeWriteMsg=warning  WriteAfterWriteMsg=warning  WriteAfterReadMsg=warning  ShowAdditionalParam=off
  Data Store Read : DataStoreRead  DataStoreName=Previous_IN
  Data Store Read1 : DataStoreRead  DataStoreName=Previous_OUT
  Data Store Write : DataStoreWrite  DataStoreName=Previous_IN
  Data Store Write1 : DataStoreWrite  DataStoreName=Previous_OUT
  Gain : Gain  Gain=-1
  Product : Product
  Product1 : Product
  Subtract : Sum  Inputs=-+
  Subtract1 : Sum
  ct : Constant
  exp(-tcycle/tau)1 : Constant  Value=0.905
  OUT : Outport
  wires:
  IN/1 -> Data Store Write/1
  Data Store Read/1 -> Product/1
  Data Store Read1/1 -> Product1/2
  ct/1 -> Subtract/1
  Subtract/1 -> Product/2
  exp(-tcycle/tau)1/1 -> Product1/1, Subtract/2
  Product/1 -> Subtract1/1
  Product1/1 -> Subtract1/2
  Subtract1/1 -> Gain/1, Data Store Write1/1
  Gain/1 -> OUT/1

== system Torque_Control_ETR07/Temperatures_Control/If Action Subsystem ==
  Action Port : ActionPort
  Constant : Constant
  Problema : Outport
  wires:
  Constant/1 -> Problema/1

== system Torque_Control_ETR07/Temperatures_Control/If Action Subsystem1 ==
  Action Port : ActionPort
  Constant : Constant  Value=0
  Ok : Outport
  wires:
  Constant/1 -> Ok/1

== system Torque_Control_ETR07/Temperatures_Control/If Action Subsystem2 ==
  Action Port : ActionPort
  Constant : Constant
  Problema : Outport
  wires:
  Constant/1 -> Problema/1

== system Torque_Control_ETR07/Temperatures_Control/If Action Subsystem3 ==
  Action Port : ActionPort
  Constant : Constant  Value=0
  OK : Outport
  wires:
  Constant/1 -> OK/1

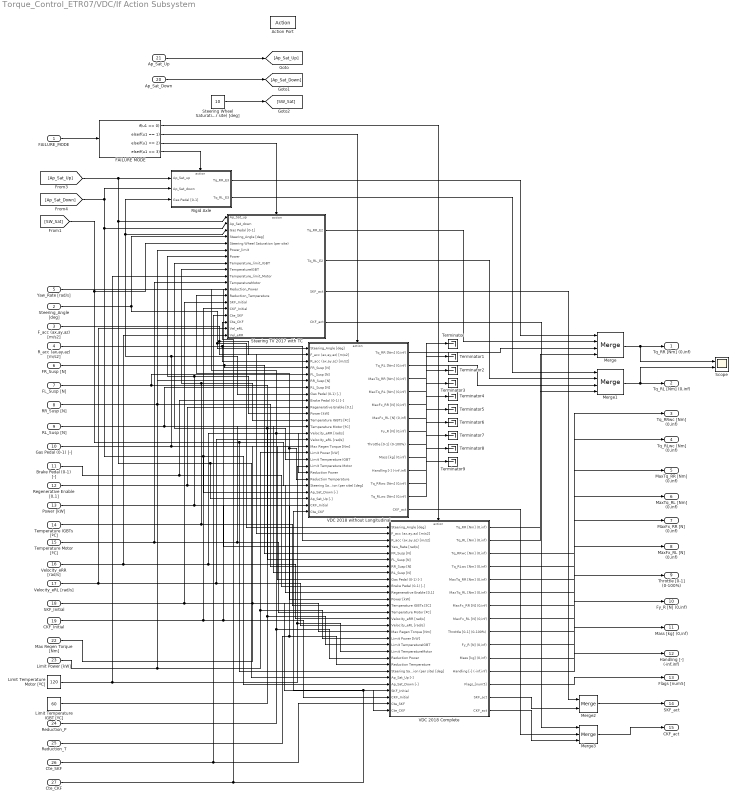
== system Torque_Control_ETR07/VDC/If Action Subsystem ==
  FAILURE_MODE : Inport
  Steering_Angle [deg] : Inport  Port=2
  F_acc (ax,ay,az) [m/s2] : Inport  Port=3
  R_acc (ax,ay,az) [m/s2] : Inport  Port=4
  Yaw_Rate [rad/s] : Inport  Port=5
  FR_Susp [N] : Inport  Port=6
  FL_Susp [N] : Inport  Port=7
  RR_Susp [N] : Inport  Port=8
  RL_Susp [N] : Inport  Port=9
  Gas Pedal (0-1) [-] : Inport  Port=10
  Brake Pedal (0-1) [-] : Inport  Port=11
  Regenerative Enable [0,1] : Inport  Port=12
  Power [kW] : Inport  Port=13
  Temperature IGBTs [ºC] : Inport  Port=14
  Temperature Motor [ºC] : Inport  Port=15
  Velocity_eRR [rad/s] : Inport  Port=16
  Velocity_eRL [rad/s] : Inport  Port=17
  SKF_Initial : Inport  Port=18
  CKF_Initial : Inport  Port=19
  Ap_Sat_Down : Inport  Port=20
  Ap_Sat_Up : Inport  Port=21
  Max Regen Torque [Nm] : Inport  Port=22
  Limit Power [kW] : Inport  Port=23
  Reduction_P : Inport  Port=24
  Reduction_T : Inport  Port=25
  Cte_SKF : Inport  Port=26
  Cte_CKF : Inport  Port=27
  Action Port : ActionPort  ActionType=then
  FAILURE MODE : If  IfExpression=u1 == 0  ElseIfExpressions=u1 == 1, u1 == 2, u1 == 3  ShowElse=off
  Limit Temperature IGBT [ºC] : Constant  Value=60
  Limit Temperature Motor [ºC] : Constant  Value=120
  Merge : Merge  Inputs=4
  Merge1 : Merge  Inputs=4
  Merge2 : Merge
  Merge3 : Merge  Inputs=3
  Rigid Axle : Subsystem  TreatAsAtomicUnit=on
  Scope : Scope  NumInputPorts=2
  Steering TV 2017 with TC : Subsystem  TreatAsAtomicUnit=on
  "Steering Wheel Saturation (per site) [deg] " : Constant  Value=10
  Terminator{,1..9} (10 alike) : Terminator
  VDC 2018 Complete : Subsystem  TreatAsAtomicUnit=on
  VDC 2018 without Longitudinal : Subsystem  TreatAsAtomicUnit=on
  Tq_RR [Nm] (0,inf) : Outport
  Tq_RL [Nm] (0,inf) : Outport  Port=2
  Tq_RRwc [Nm] (0,inf) : Outport  Port=3
  Tq_RLwc [Nm] (0,inf) : Outport  Port=4
  MaxTq_RR [Nm] (0,inf) : Outport  Port=5
  MaxTq_RL [Nm] (0,inf) : Outport  Port=6
  MaxFx_RR [N] (0,inf) : Outport  Port=7
  MaxFx_RL [N] (0,inf) : Outport  Port=8
  Throttle [0-1] (0-100%) : Outport  Port=9
  Fy_R [N] (0,inf) : Outport  Port=10
  Mass [kg] (0,inf) : Outport  Port=11
  Handling [-] (-inf,inf) : Outport  Port=12
  Flags [num5] : Outport  Port=13
  SKF_act : Outport  Port=14
  CKF_act : Outport  Port=15
  wires:
  RL_Susp [N]/1 -> VDC 2018 Complete/8(RL_Susp [N]), VDC 2018 without Longitudinal/7(RL_Susp [N])
  R_acc (ax,ay,az) [m/s2]/1 -> VDC 2018 Complete/3(R_acc (ax,ay,az) [m/s2]), VDC 2018 without Longitudinal/3(R_acc (ax,ay,az) [m/s2])
  Steering TV 2017 with TC/4(CKF_act) -> Merge3/1
  Cte_SKF/1 -> Steering TV 2017 with TC/16(Cte_SKF), VDC 2018 Complete/28(Cte_SKF)
  VDC 2018 without Longitudinal/13(CKF_act) -> Merge3/2
  Steering TV 2017 with TC/3(SKF_act) -> Merge2/1
  Merge3/1 -> CKF_act/1
  VDC 2018 Complete/10(Fy_R [N] (0,inf)) -> Fy_R [N] (0,inf)/1
  Yaw_Rate [rad/s]/1 -> VDC 2018 Complete/4(Yaw_Rate [rad/s])
  VDC 2018 without Longitudinal/2(Tq_RL [Nm] (0,inf)) -> Merge1/3
  Merge2/1 -> SKF_act/1
  VDC 2018 Complete/15(CKF_act) -> Merge3/3
  VDC 2018 without Longitudinal/12(Tq_RLwc [Nm] (0,inf)) -> Terminator9/1
  VDC 2018 without Longitudinal/9(Mass [kg] (0,inf)) -> Terminator6/1
  Gas Pedal (0-1) [-]/1 -> VDC 2018 Complete/9(Gas Pedal (0-1) [-]), Steering TV 2017 with TC/3(Gas Pedal [0-1]), Rigid Axle/3(Gas Pedal [0-1]), VDC 2018 without Longitudinal/8(Gas Pedal (0-1) [-])
  Limit Temperature IGBT [ºC]/1 -> VDC 2018 without Longitudinal/18(Limit Temperature IGBT), Steering TV 2017 with TC/8(Temperature_limit_IGBT), VDC 2018 Complete/19(Limit TemperatureIGBT)
  SKF_Initial/1 -> VDC 2018 Complete/26(SKF_Initial), Steering TV 2017 with TC/14(SKF_Initial)
  Cte_CKF/1 -> Steering TV 2017 with TC/17(Cte_CKF), VDC 2018 without Longitudinal/26(Cte_CKF), VDC 2018 Complete/29(Cte_CKF)
  VDC 2018 Complete/13(Flags_[num5]) -> Flags [num5]/1
  VDC 2018 without Longitudinal/4(MaxTq_RL [Nm] (0,inf)) -> Terminator1/1
  VDC 2018 without Longitudinal/11(Tq_RRwc [Nm] (0,inf)) -> Terminator8/1
  Steering_Angle [deg]/1 -> VDC 2018 Complete/1(Steering_Angle [deg]), VDC 2018 without Longitudinal/1(Steering_Angle [deg]), Steering TV 2017 with TC/4(Steering_Angle [deg])
  Reduction_P/1 -> Steering TV 2017 with TC/12(Reduction_Power), VDC 2018 without Longitudinal/20(Reduction Power), VDC 2018 Complete/21(Reduction Power)
  VDC 2018 without Longitudinal/3(MaxTq_RR [Nm] (0,inf)) -> Terminator/1
  Brake Pedal (0-1) [-]/1 -> VDC 2018 Complete/10(Brake Pedal (0-1) [-]), VDC 2018 without Longitudinal/9(Brake Pedal (0-1) [-])
  VDC 2018 without Longitudinal/6(MaxFx_RL [N] (0,inf)) -> Terminator3/1
  VDC 2018 Complete/11(Mass [kg] (0,inf)) -> Mass [kg] (0,inf)/1
  Velocity_eRR [rad/s]/1 -> Steering TV 2017 with TC/19(Vel_eRR), VDC 2018 without Longitudinal/14(Velocity_eRR [rad/s]), VDC 2018 Complete/15(Velocity_eRR [rad/s])
  VDC 2018 without Longitudinal/8(Throttle [0-1] (0-100%)) -> Terminator5/1
  F_acc (ax,ay,az) [m/s2]/1 -> VDC 2018 Complete/2(F_acc (ax,ay,az) [m/s2]), VDC 2018 without Longitudinal/2(F_acc (ax,ay,az) [m/s2])
  VDC 2018 without Longitudinal/7(Fy_R [N] (0,inf)) -> Terminator4/1
  Ap_Sat_Up/1 -> [Ap_Sat_Up]
  Merge/1 -> Scope/1, Tq_RR [Nm] (0,inf)/1
  VDC 2018 Complete/12(Handling [-] (-inf,inf)) -> Handling [-] (-inf,inf)/1
  VDC 2018 without Longitudinal/1(Tq_RR [Nm] (0,inf)) -> Merge/3
  Max Regen Torque [Nm]/1 -> VDC 2018 without Longitudinal/16(Max Regen Torque [Nm]), VDC 2018 Complete/17(Max Regen Torque [Nm])
  FR_Susp [N]/1 -> VDC 2018 without Longitudinal/4(FR_Susp [N]), VDC 2018 Complete/5(FR_Susp [N])
  VDC 2018 Complete/4(Tq_RLwc [Nm] (0,inf)) -> Tq_RLwc [Nm] (0,inf)/1
  VDC 2018 without Longitudinal/5(MaxFx_RR [N] (0,inf)) -> Terminator2/1
  VDC 2018 Complete/3(Tq_RRwc [Nm] (0,inf)) -> Tq_RRwc [Nm] (0,inf)/1
  Limit Temperature Motor [ºC]/1 -> VDC 2018 without Longitudinal/19(Limit Temperature Motor), VDC 2018 Complete/20(Limit TemperatureMotor), Steering TV 2017 with TC/10(Temperature_limit_Motor)
  Rigid Axle/2(Tq_RL_E3) -> Merge1/1
  VDC 2018 Complete/9(Throttle [0-1] (0-100%)) -> Throttle [0-1] (0-100%)/1
  Reduction_T/1 -> Steering TV 2017 with TC/13(Reduction_Temperature), VDC 2018 without Longitudinal/21(Reduction Temperature), VDC 2018 Complete/22(Reduction Temperature)
  [Ap_Sat_Up] -> Rigid Axle/1("Ap_Sat_up "), VDC 2018 Complete/24(Ap_Sat_Up [-]), VDC 2018 without Longitudinal/24(Ap_Sat_Up [-]), Steering TV 2017 with TC/1("Ap_Sat_up ")
  Temperature Motor [ºC]/1 -> VDC 2018 without Longitudinal/13(Temperature Motor [ºC]), VDC 2018 Complete/14(Temperature Motor [ºC]), Steering TV 2017 with TC/11(TemperatureMotor)
  VDC 2018 Complete/6(MaxTq_RL [Nm] (0,inf)) -> MaxTq_RL [Nm] (0,inf)/1
  CKF_Initial/1 -> Steering TV 2017 with TC/15(CKF_Initial), VDC 2018 without Longitudinal/25(CKF_Initial), VDC 2018 Complete/27(CKF_Initial)
  Velocity_eRL [rad/s]/1 -> Steering TV 2017 with TC/18(Vel_eRL), VDC 2018 without Longitudinal/15(Velocity_eRL [rad/s]), VDC 2018 Complete/16(Velocity_eRL [rad/s])
  VDC 2018 Complete/7(MaxFx_RR [N] (0,inf)) -> MaxFx_RR [N] (0,inf)/1
  VDC 2018 Complete/5(MaxTq_RR [Nm] (0,inf)) -> MaxTq_RR [Nm] (0,inf)/1
  VDC 2018 Complete/1(Tq_RR [Nm] (0,inf)) -> Merge/4
  Power [kW]/1 -> Steering TV 2017 with TC/7(Power), VDC 2018 without Longitudinal/11(Power [kW]), VDC 2018 Complete/12(Power [kW])
  VDC 2018 Complete/2(Tq_RL [Nm] (0,inf)) -> Merge1/4
  RR_Susp [N]/1 -> VDC 2018 without Longitudinal/6(RR_Susp [N]), VDC 2018 Complete/7(RR_Susp [N])
  VDC 2018 without Longitudinal/10(Handling [-] (-inf,inf)) -> Terminator7/1
  [SW_Sat] -> Steering TV 2017 with TC/5("Steering Wheel Saturation (per site) "), VDC 2018 Complete/23(Steering Saturation (per site) [deg]), VDC 2018 without Longitudinal/22(Steering Saturation (per site) [deg])
  Regenerative Enable [0,1]/1 -> VDC 2018 Complete/11(Regenerative Enable [0,1]), VDC 2018 without Longitudinal/10(Regenerative Enable [0,1])
  Limit Power [kW]/1 -> Steering TV 2017 with TC/6(Power_limit), VDC 2018 without Longitudinal/17(Limit Power [kW]), VDC 2018 Complete/18(Limit Power [kW])
  FAILURE MODE/3 -> Steering TV 2017 with TC/Action
  VDC 2018 Complete/14(SKF_act) -> Merge2/2
  [Ap_Sat_Down] -> VDC 2018 Complete/25(Ap_Sat_Down [-]), VDC 2018 without Longitudinal/23(Ap_Sat_Down [-]), Steering TV 2017 with TC/2(Ap_Sat_down), Rigid Axle/2(Ap_Sat_down)
  Steering TV 2017 with TC/2(Tq_RL_E2) -> Merge1/2
  Temperature IGBTs [ºC]/1 -> VDC 2018 Complete/13(Temperature IGBTs [ºC]), Steering TV 2017 with TC/9(TemperatureIGBT), VDC 2018 without Longitudinal/12(Temperature IGBTs [ºC])
  "Steering Wheel Saturation (per site) [deg] "/1 -> [SW_Sat]
  VDC 2018 Complete/8(MaxFx_RL [N] (0,inf)) -> MaxFx_RL [N] (0,inf)/1
  FL_Susp [N]/1 -> VDC 2018 without Longitudinal/5(FL_Susp [N]), VDC 2018 Complete/6(FL_Susp [N])
  Ap_Sat_Down/1 -> [Ap_Sat_Down]
  Merge1/1 -> Scope/2, Tq_RL [Nm] (0,inf)/1
  FAILURE MODE/4 -> Rigid Axle/Action
  Rigid Axle/1(Tq_RR_E3) -> Merge/1
  Steering TV 2017 with TC/1(Tq_RR_E2) -> Merge/2
  FAILURE_MODE/1 -> FAILURE MODE/1
  FAILURE MODE/1 -> VDC 2018 Complete/Action
  FAILURE MODE/2 -> VDC 2018 without Longitudinal/Action

== system Torque_Control_ETR07/VDC/Regeneration_Enable ==
  Cell_Temp_ºC : Inport
  Brake_0_to_1 : Inport  Port=2
  Velocity_RR : Inport  Port=3
  Velocity_RL : Inport  Port=4
  Add : Sum
  BRAKE_THRESHOLD : Constant  Value=0.2
  Braking : Subsystem  TreatAsAtomicUnit=on
  "BypassDecision " : Subsystem  TreatAsAtomicUnit=on
  Constant : Constant  Value=2
  Data Store Memory : DataStoreMemory  DataStoreName=R  ReadBeforeWriteMsg=warning  WriteAfterWriteMsg=warning  WriteAfterReadMsg=warning  ShowAdditionalParam=off
  Data Store Read : DataStoreRead  DataStoreName=R
  Data Store Write : DataStoreWrite  DataStoreName=R
  Divide : Product  Inputs=*/
  If : If  NumInputs=2  IfExpression=(u1>0)&(u2>0)
  If1 : If  NumInputs=2  IfExpression=u1 > u2
  Merge : Merge
  Merge1 : Merge
  Not-Braking : Subsystem  TreatAsAtomicUnit=on
  NotEnabled : Subsystem  TreatAsAtomicUnit=on
  "Zero " : Constant  Value=0
  Regeneration_Enable : Outport
  Regeneration_Enable_Abs : Outport  Port=2
  Mean_Speed : Outport  Port=3
  wires:
  BRAKE_THRESHOLD/1 -> If1/2
  Brake_0_to_1/1 -> If1/1
  If1/1 -> Braking/Action
  If1/2 -> Not-Braking/Action
  Cell_Temp_ºC/1 -> Not-Braking/1(Cell_Temp_ºC)
  Data Store Read/1 -> Braking/1(Latched), Not-Braking/2(Prev_State)
  Not-Braking/2(Temp_Enable) -> Regeneration_Enable_Abs/1, Data Store Write/1
  Braking/1(Enable) -> Merge/1
  Not-Braking/1(Enable) -> Merge/2
  Merge/1 -> "BypassDecision "/1(In1)
  "BypassDecision "/1(Out1) -> Merge1/2
  Merge1/1 -> Regeneration_Enable/1
  NotEnabled/1(Out1) -> Merge1/1
  Velocity_RR/1 -> Add/1, If/1
  Velocity_RL/1 -> Add/2, If/2
  If/1 -> "BypassDecision "/Action
  If/2 -> NotEnabled/Action
  "Zero "/1 -> NotEnabled/1(In1)
  Add/1 -> Divide/1
  Divide/1 -> Mean_Speed/1
  Constant/1 -> Divide/2

== system Torque_Control_ETR07/VDC/TEST_MODE_IN ==
  Workshop_Mode_Enable : Inport
  Suspension_FR_N_in : Inport  Port=2
  Suspension_FL_N_in : Inport  Port=3
  Suspension_RL_N_in : Inport  Port=4
  Suspension_RR_N_in : Inport  Port=5
  BYPASS : Subsystem  TreatAsAtomicUnit=on
  If : If  IfExpression=u1 == 1
  Merge{,1..3} (4 alike) : Merge
  TEST_CONSTANTS : Subsystem  TreatAsAtomicUnit=on
  Suspension_FR_N_out : Outport
  Suspension_FL_N_out : Outport  Port=2
  Suspension_RR_N_out : Outport  Port=3
  Suspension_RL_N_out : Outport  Port=4
  wires:
  Suspension_FR_N_in/1 -> BYPASS/1(In1)
  Suspension_FL_N_in/1 -> BYPASS/2(In2)
  Suspension_RR_N_in/1 -> BYPASS/3(In3)
  Suspension_RL_N_in/1 -> BYPASS/4(In4)
  Merge/1 -> Suspension_FR_N_out/1
  Merge1/1 -> Suspension_FL_N_out/1
  Merge2/1 -> Suspension_RR_N_out/1
  Merge3/1 -> Suspension_RL_N_out/1
  BYPASS/1(Out1) -> Merge/1
  BYPASS/2(Out2) -> Merge1/1
  BYPASS/3(Out3) -> Merge2/1
  BYPASS/4(Out4) -> Merge3/1
  Workshop_Mode_Enable/1 -> If/1
  If/2 -> BYPASS/Action
  If/1 -> TEST_CONSTANTS/Action
  TEST_CONSTANTS/4(Out4) -> Merge3/2
  TEST_CONSTANTS/3(Out3) -> Merge2/2
  TEST_CONSTANTS/2(Out2) -> Merge1/2
  TEST_CONSTANTS/1(Out1) -> Merge/2

== system Torque_Control_ETR07/VDC/WORKSHOP_MODE_RESTRICTIONS ==
  Workshop_Mode_Enable : Inport
  Torque_R_in : Inport  Port=2
  Torque_L_in : Inport  Port=3
  BYPASS : Subsystem  TreatAsAtomicUnit=on
  If : If  IfExpression=u1 == 1
  Merge : Merge
  Merge1 : Merge
  Saturation : Saturate  UpperLimit=145  LowerLimit=-70
  Saturation1 : Saturate  UpperLimit=145  LowerLimit=-70
  "Torque_Reduction " : Subsystem  TreatAsAtomicUnit=on
  Torque_L_out : Outport
  Torque_R_out : Outport  Port=2
  wires:
  If/2 -> BYPASS/Action
  If/1 -> "Torque_Reduction "/Action
  Workshop_Mode_Enable/1 -> If/1
  Torque_R_in/1 -> BYPASS/1(In1), "Torque_Reduction "/1(In1)
  Torque_L_in/1 -> "Torque_Reduction "/2(In2), BYPASS/2(In2)
  BYPASS/1(Out1) -> Merge/1
  BYPASS/2(Out2) -> Merge1/2
  "Torque_Reduction "/1(Out1) -> Merge/2
  "Torque_Reduction "/2(Out2) -> Merge1/1
  Merge/1 -> Saturation/1
  Merge1/1 -> Saturation1/1
  Saturation/1 -> Torque_R_out/1
  Saturation1/1 -> Torque_L_out/1

== system Torque_Control_ETR07/Accumulator Power/PowerLimitDetection/LimitReached ==
  Action Port : ActionPort  ActionType=then
  Constant : Constant
  "Out " : Outport
  wires:
  Constant/1 -> "Out "/1

== system Torque_Control_ETR07/Accumulator Power/PowerLimitDetection/OK_OrLatch ==
  IN : Inport
  Action Port : ActionPort  ActionType=else
  If : If  IfExpression=(u1>0)
  Latched Error : Subsystem  TreatAsAtomicUnit=on
  Merge : Merge
  OK : Subsystem  TreatAsAtomicUnit=on
  Out 1 : Outport
  wires:
  IN/1 -> If/1
  If/1 -> Latched Error/Action
  If/2 -> OK/Action
  Latched Error/1("Out ") -> Merge/1
  OK/1("Out ") -> Merge/2
  Merge/1 -> Out 1/1

== system Torque_Control_ETR07/Calculate Current Conversion/KT_L_TORKY/Bypass ==
  In1 : Inport
  In2 : Inport  Port=2
  Action Port : ActionPort  ActionType=then
  Out1 : Outport
  Out2 : Outport  Port=2
  wires:
  In1/1 -> Out1/1
  In2/1 -> Out2/1

== system Torque_Control_ETR07/Calculate Current Conversion/KT_L_TORKY/Bypass_Torque ==
  In1 : Inport
  Action Port : ActionPort  ActionType=else
  Out1 : Outport
  wires:
  In1/1 -> Out1/1

== system Torque_Control_ETR07/Calculate Current Conversion/KT_L_TORKY/Is_Zero ==
  In1 : Inport
  Action Port : ActionPort  ActionType=then
  Out1 : Outport
  wires:
  In1/1 -> Out1/1

== system Torque_Control_ETR07/Calculate Current Conversion/KT_L_TORKY/Negative ==
  In1 : Inport
  In2 : Inport  Port=2
  Action Port : ActionPort  ActionType=else
  Gain : Gain  Gain=-1
  Gain1 : Gain  Gain=-1
  Out1 : Outport
  Out2 : Outport  Port=2
  wires:
  In2/1 -> Gain1/1
  In1/1 -> Gain/1
  Gain/1 -> Out1/1
  Gain1/1 -> Out2/1

== system Torque_Control_ETR07/Calculate Current Conversion/KT_R_EMY/Bypass ==
  In1 : Inport
  In2 : Inport  Port=2
  Action Port : ActionPort  ActionType=then
  Out1 : Outport
  Out2 : Outport  Port=2
  wires:
  In1/1 -> Out1/1
  In2/1 -> Out2/1

== system Torque_Control_ETR07/Calculate Current Conversion/KT_R_EMY/Bypass_Torque ==
  In1 : Inport
  Action Port : ActionPort  ActionType=else
  Out1 : Outport
  wires:
  In1/1 -> Out1/1

== system Torque_Control_ETR07/Calculate Current Conversion/KT_R_EMY/Is_Zero ==
  In1 : Inport
  Action Port : ActionPort  ActionType=then
  Out1 : Outport
  wires:
  In1/1 -> Out1/1

== system Torque_Control_ETR07/Calculate Current Conversion/KT_R_EMY/Negative ==
  In1 : Inport
  In2 : Inport  Port=2
  Action Port : ActionPort  ActionType=else
  Gain : Gain  Gain=-1
  Gain1 : Gain  Gain=-1
  Out1 : Outport
  Out2 : Outport  Port=2
  wires:
  In2/1 -> Gain1/1
  In1/1 -> Gain/1
  Gain/1 -> Out1/1
  Gain1/1 -> Out2/1

== system Torque_Control_ETR07/SAFETY BLOCK/APPS_IMPLAUSIBILITY/Imp ==
  Action Port : ActionPort  ActionType=then
  Constant : Constant  Value=0  OutDataTypeStr=boolean
  Out1 : Outport
  wires:
  Constant/1 -> Out1/1  "Boolean"

== system Torque_Control_ETR07/SAFETY BLOCK/APPS_IMPLAUSIBILITY/Not Imp ==
  Action Port : ActionPort  ActionType=else
  Constant : Constant  OutDataTypeStr=boolean
  Out1 : Outport
  wires:
  Constant/1 -> Out1/1  "Boolean"

== system Torque_Control_ETR07/SAFETY BLOCK/BRAKE_IMPLAUSIBILITY/If Action Subsystem2 ==
  Action Port : ActionPort  ActionType=then
  Constant : Constant
  Out1 : Outport
  wires:
  Constant/1 -> Out1/1

== system Torque_Control_ETR07/SAFETY BLOCK/BRAKE_IMPLAUSIBILITY/If Action Subsystem3 ==
  Action Port : ActionPort  ActionType=else
  Constant : Constant  Value=0
  Out1 : Outport
  wires:
  Constant/1 -> Out1/1

== system Torque_Control_ETR07/SAFETY BLOCK/BRAKE_IMPLAUSIBILITY/Imp Memo1 ==
  Action Port : ActionPort  ActionType=then
  Constant : Constant  Value=0  OutDataTypeStr=boolean
  Out1 : Outport
  wires:
  Constant/1 -> Out1/1  "Boolean"

== system Torque_Control_ETR07/SAFETY BLOCK/BRAKE_IMPLAUSIBILITY/Imp1 ==
  Action Port : ActionPort  ActionType=then
  Constant : Constant  Value=0  OutDataTypeStr=boolean
  Out1 : Outport
  wires:
  Constant/1 -> Out1/1  "Boolean"

== system Torque_Control_ETR07/SAFETY BLOCK/BRAKE_IMPLAUSIBILITY/Not Imp Memo1 ==
  Action Port : ActionPort  ActionType=else
  Constant : Constant  OutDataTypeStr=boolean
  Out1 : Outport
  wires:
  Constant/1 -> Out1/1  "Boolean"

== system Torque_Control_ETR07/SAFETY BLOCK/BRAKE_IMPLAUSIBILITY/Not Imp1 ==
  Action Port : ActionPort  ActionType=else
  Constant : Constant  OutDataTypeStr=boolean
  Out1 : Outport
  wires:
  Constant/1 -> Out1/1  "Boolean"

== system Torque_Control_ETR07/VDC/If Action Subsystem/Rigid Axle ==
  "Ap_Sat_up " : Inport
  Ap_Sat_down : Inport  Port=2
  Gas Pedal [0-1] : Inport  Port=3
  Action Port : ActionPort  ActionType=elseif
  Accelerating : Subsystem
  Torque_RL [Nm] : Constant  Value=60
  Torque_RR [Nm] : Constant  Value=60
  Tq_RR_E3 : Outport
  Tq_RL_E3 : Outport  Port=2
  wires:
  Gas Pedal [0-1]/1 -> Accelerating/1(Ap)
  "Ap_Sat_up "/1 -> Accelerating/2("Ap_Sat_up ")
  Ap_Sat_down/1 -> Accelerating/3(Ap_Sat_down)
  Accelerating/1("Tq_RR ") -> Tq_RR_E3/1
  Accelerating/2(Tq_RL) -> Tq_RL_E3/1
  Torque_RR [Nm]/1 -> Accelerating/4(Tq_RR)
  Torque_RL [Nm]/1 -> Accelerating/5("Tq_RL ")
